simulink model "minimalist10"  (Simulink 7.4)
settings: Solver=FixedStepDiscrete  StartTime=0.0  StopTime=inf  RelTol=1e-3  SampleTimeConstraint=STIndependent
PreLoadFcn:
  | RTWConfigurationCB('preloadfcn', bdroot);
PostLoadFcn:
  | mpc555rt_switch_target(gcs,'auto')
libraries: mpc555drivers x3
CloseFcn:
  | rtwprivate ssgencode ModelCloseRequest foo
settings Model: Creator=The MathWorks Inc.  LastModifiedBy=autopilot
settings DataIOCC: LimitDataPoints=off  SignalLoggingName=sigsOut
settings OptimizationCC: InlineParams=on  InlineInvariantSignals=on  EnforceIntegerDowncast=off  ZeroExternalMemoryAtStartup=off  ZeroInternalMemoryAtStartup=off  InitFltsAndDblsToZero=on  NoFixptDivByZeroProtection=on  OptimizeModelRefInitCode=on  LifeSpan=1
settings DebuggingCC: SaveWithParameterizedLinksMsg=none  SignalResolutionControl=TryResolveAllWithWarning  SolverPrmCheckMsg=none  MultiTaskDSMMsg=warning  MultiTaskCondExecSysMsg=none  UnderSpecifiedDataTypeMsg=error  StrictBusMsg=ErrorLevel1
settings HardwareCC: ProdEndianess=BigEndian  ProdHWDeviceType=Motorola PowerPC
settings RTWCC: SystemTargetFile=mpc555rt.tlc  TemplateMakefile=mpc555rt.tmf  Description=Target Support Package (for use with Freescale MPC5xx) (real-time)  ProcessScript=mpc555rt_make_rtw_hook
settings CodeAppCC: IgnoreCustomStorageClasses=off
settings STFCustomTargetCC: TargetFcnLib=ansi_tfl_tmw.mat  TargetLibSuffix=.a  TargetPreCompLibLocation=C:\Program Files\MATLAB\R2009b\toolbox\rtw\targets\mpc555dk\drivers\lib\CODE_WARRIOR  IncludeMdlTerminateFcn=off  CombineOutputUpdateFcns=on  ERTCustomFileBanners=on  SupportAbsoluteTime=off  SupportNonFinite=off  SupportComplex=off  SupportContinuousTime=off  SupportNonInlinedSFcns=off  CPPClassGenCompliant=on  SystemTargetFile=mpc555rt.tlc
settings ERTTargetCC: TargetFcnLib=ansi_tfl_tmw.mat  TargetPreCompLibLocation=C:\Program Files\MATLAB\R2009b\toolbox\rtw\targets\mpc555dk\drivers\lib\CODE_WARRIOR  MultiwordLength=2048  ParMdlRefBuildCompliant=off  CompOptLevelCompliant=off  IncludeMdlTerminateFcn=off  ERTFirstTimeCompliant=off  SupportAbsoluteTime=off  SupportNonFinite=off  SupportComplex=off  ModelStepFunctionPrototypeControlCompliant=off  ExtModeMexFile=MPC5xxExternalModeOpen  ExtModeIntrfLevel=Level2 - Open  ERTCustomFileTemplate=example_file_process.tlc  ConvertIfToSwitch=off
settings CustomProperty: DataType=RTWOptions_EnumType__toolbox_rtw_targets_mpc555dk_mpc555dk_mpc555rt_1MPC555_OPTIMIZATION_SWITCH  Value=speed
settings EnumStrPairs: String=speed

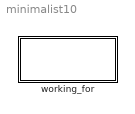
== system minimalist10 ==
  working_for : Subsystem  InitFcn=|
      | % START RTW CONFIGURATION CODE %
      | RTWConfigurationCB('rtw_target_initfcn',gcb);
      | % END RTW CONFIGURATION CODE %

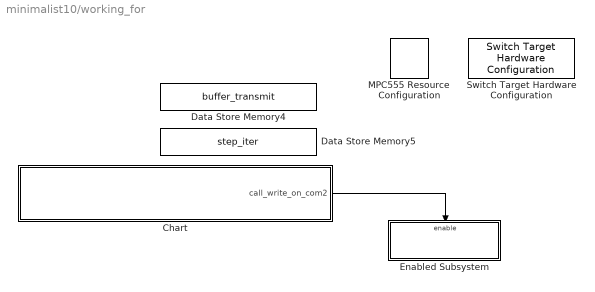
== system minimalist10/working_for ==
  Chart : Stateflow chart  TreatAsAtomicUnit=on
      settings: RTWSystemCode=Inline
  Data Store Memory4 : DataStoreMemory  DataStoreName=buffer_transmit  InitialValue=[65 66 67 68 69 70 71 72 13 10]  DataType=uint8  OutDataType=fixdt(1, 16)  OutScaling=2^0  OutDataTypeStr=uint8
  Data Store Memory5 : DataStoreMemory  DataStoreName=step_iter  DataType=uint8  OutDataType=fixdt(1, 16)  OutScaling=2^0  OutDataTypeStr=uint8
  Enabled Subsystem : Subsystem  TreatAsAtomicUnit=on
  MPC555 Resource Configuration : mpc555drivers/MPC555 Resource Configuration  Tag=RTW CONFIGURATION BLOCK  Priority=-100000  SystemSampleTime=-1  oldParentName=minimalist10/working_for  oldBlockName=|
      | minimalist10/working_for/MPC555
      | Resource
      | Configuration
  Switch Target Hardware Configuration : mpc555drivers/Utilities/Switch Target Hardware Configuration  SystemSampleTime=-1
  wires:
  Chart/1(call_write_on_com2) -> Enabled Subsystem/Enable

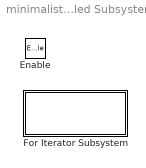
== system minimalist10/working_for/Enabled Subsystem ==
  Enable : EnablePort
  For Iterator Subsystem : Subsystem  Priority=1  TreatAsAtomicUnit=on
      settings: RTWSystemCode=Inline

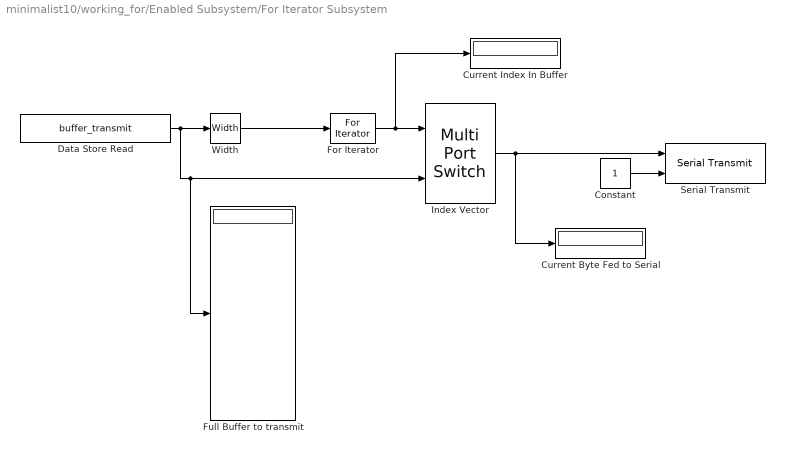
== system minimalist10/working_for/Enabled Subsystem/For Iterator Subsystem ==
  Constant : Constant  OutDataTypeMode=uint32  OutDataType=fixdt(1, 16)  OutScaling=2^0  OutDataTypeStr=uint32  SampleTime=-1
  Current Byte Fed to Serial : Display
  Current Index In Buffer : Display
  Data Store Read : DataStoreRead  DataStoreName=buffer_transmit  SampleTime=-1
  For Iterator : ForIterator  IterationSource=external
  Full Buffer to transmit : Display
  Index Vector : MultiPortSwitch  Inputs=1  OutDataType=fixdt(1, 16)  OutScaling=2^0
  Serial Transmit : mpc555drivers/Serial Communications Interface (SCI)/Serial Transmit  module=1  show_length=on  show_num_sent=off  T=-1
  Width : Width
  wires:
  For Iterator/1 -> Index Vector/1, Current Index In Buffer/1
  Index Vector/1 -> Current Byte Fed to Serial/1, Serial Transmit/1
  Data Store Read/1 -> Width/1, Index Vector/2, Full Buffer to transmit/1
  Width/1 -> For Iterator/1
  Constant/1 -> Serial Transmit/2

== stateflow chart working_for/Chart ==
  state STEP01
    call_write_on_com2=1;
    step_iter = step_iter + 1;
  state STEP02
    call_write_on_com2=0;
  STEP01 -> STEP02 [order 2] : [step_iter>=10]
  STEP01 -> STEP01 [order 1] : [step_iter<10]
  (default) -> STEP01
  data: step_iter data_store_memory double; call_write_on_com2 output uint8
